simulink model "p5_data_series_using_nth_order_forward_predictor"  (R2023a)
settings: Solver=VariableStepAuto  StartTime=0.0  StopTime=500000  RelTol=1e-3
libraries: dsplp x1, dspsrcs4 x1
settings Model: Creator=The MathWorks, Inc.  LastModifiedBy=rachi
settings SolverCC: MaxZcPerStep=1
settings DataIOCC: ReturnWorkspaceOutputs=off
settings DebuggingCC: UnconnectedInputMsg=warning  UnconnectedOutputMsg=warning  UnconnectedLineMsg=warning
settings ModelReferenceCC: EnableRefExpFcnMdlSchedulingChecks=on
settings RTWCC: DLArmComputeVersion=19.05

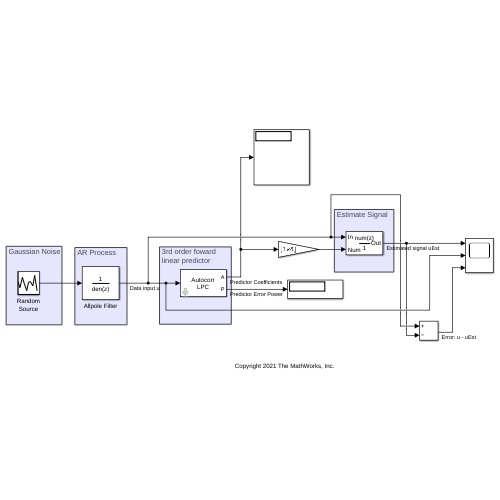
[thumbnail: Simulink's stored preview of the top-level diagram]
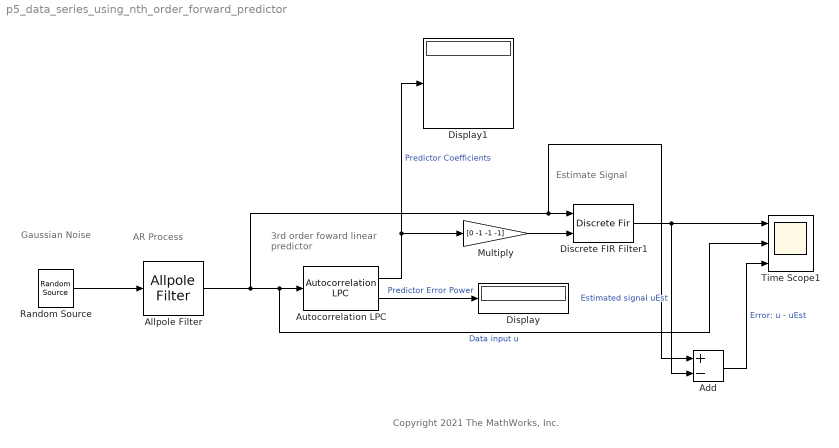
== system p5_data_series_using_nth_order_forward_predictor ==
  note: Estimate Signal
  note: 3rd order foward
      | linear predictor
  note: AR Process
  note: Gaussian Noise
  note: Copyright 2021 The MathWorks, Inc.
  Add : Sum  Inputs=+-
  Allpole Filter : AllpoleFilter  Coefficients=[1 0.5 1/3 0.25 1/5 1/6]
  Autocorrelation LPC : dsplp/Autocorrelation LPC  lpcCoeffOutFcn=A  lpcOutP=on  inherit_prediction_order=off  order=3
  Discrete FIR Filter1 : DiscreteFir  CoefSource=Input port  Coefficients=[1 0.5 1/3 0.25]
      settings: InputPortMap=u0,u1
  Display : Display
  Display1 : Display
  Multiply : Gain  Gain=[0 -1 -1 -1]
  Random Source : dspsrcs4/Random Source  SrcType=Gaussian  NormMethod=Ziggurat  CltLength=12  MinVal=0  MaxVal=0.1  MeanVal=0  VarVal=0.001  RepMode=Not repeatable  rawSeed=1  IsInherit=off  SampMode=Discrete  SampTime=0.1  SampFrame=50000  DataType=Double  OutComplex=Real  OutputFrames=off
  Time Scope1 : Scope  NumInputPorts=3
  wires:
  Random Source/1 -> Allpole Filter/1
  Allpole Filter/1 -> Add/1, Discrete FIR Filter1/1, Autocorrelation LPC/1, Time Scope1/2  "Data input u"
  Autocorrelation LPC/1 -> Multiply/1, Display1/1  "Predictor Coefficients"
  Discrete FIR Filter1/1 -> Add/2, Time Scope1/1  "Estimated signal uEst"
  Autocorrelation LPC/2 -> Display/1  "Predictor Error Power"
  Multiply/1 -> Discrete FIR Filter1/2
  Add/1 -> Time Scope1/3  "Error: u - uEst"
